simulink subsystem "VehicleEOMRef_Simp"  (R2022b)
settings: Solver=VariableStepAuto  StartTime=0.0  StopTime=10.0  RelTol=1e-3
undefined symbols (not defined in the file): Accel_bIi, Asensed_bIb, Newton, Omeg_BIb, OmegDtI_BIb, Pos_bii, Q_i2b, Raphson, SimIn, SimPar, Vel_bIi
libraries: libAxisTransformations x9, libMathOperations x9, libGeodesy x1, libKinematicalEquations x1
settings Model: Creator=drhill  LastModifiedBy=macheson
settings SolverCC: AlgebraicLoopSolver=TrustRegion
settings DebuggingCC: UnconnectedInputMsg=warning  UnconnectedOutputMsg=warning  UnconnectedLineMsg=warning  SFMachineParentedDataDiag=warning
settings ModelReferenceCC: EnableRefExpFcnMdlSchedulingChecks=on
settings RTWCC: DLArmComputeVersion=19.05

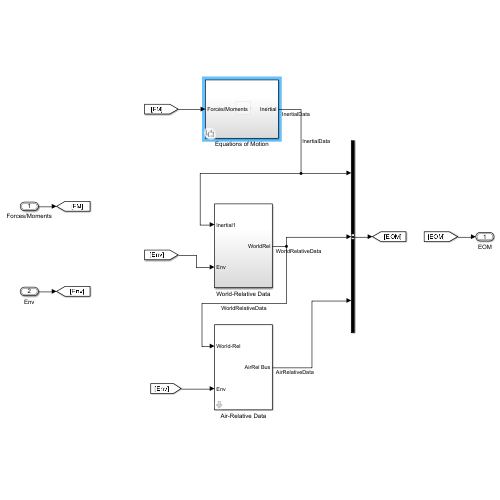
[thumbnail: Simulink's stored preview of the top-level diagram]
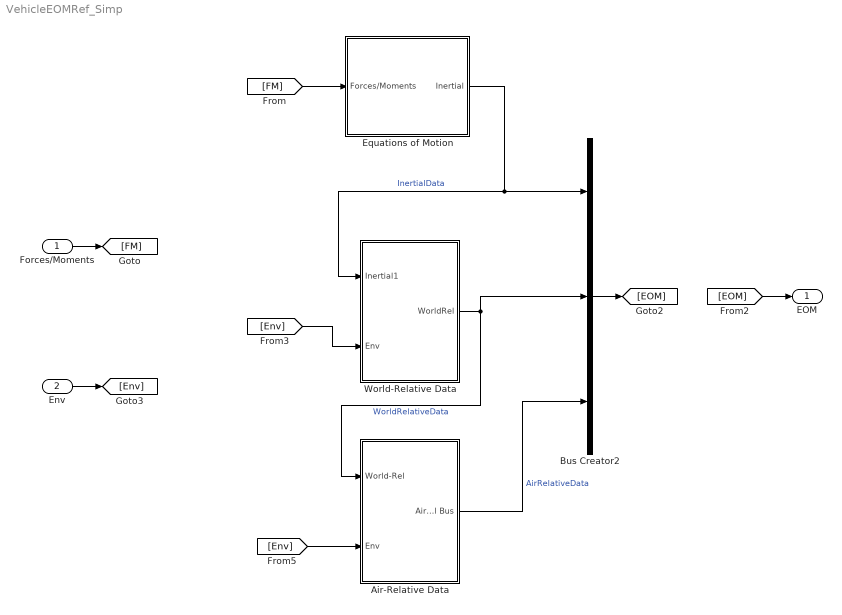
== system VehicleEOMRef_Simp ==
  Forces/Moments : Inport  OutDataTypeStr=Bus: ForceMomentBus
  Env : Inport  Port=2  OutDataTypeStr=Bus: EnvironmentBus
  Air-Relative Data : Subsystem  mask(Air-Relative Data (template)){}
      mask help: Template for common air-relative data.
  Bus Creator2 : BusCreator  Inputs=3  OutDataTypeStr=Bus: EomBus
  Equations of Motion : Subsystem  Variant=on  VariantControl=Variant1
  World-Relative Data : Subsystem
  EOM : Outport  OutDataTypeStr=Bus: EomBus
  wires:
  World-Relative Data/1(WorldRel) -> Air-Relative Data/1(World-Rel), Bus Creator2/2  "WorldRelativeData"
  Equations of Motion/1(Inertial) -> Bus Creator2/1, World-Relative Data/1(Inertial1)  "InertialData"
  Air-Relative Data/1(AirRel Bus) -> Bus Creator2/3  "AirRelativeData"
  [Env] -> Air-Relative Data/2(Env)
  [Env] -> World-Relative Data/2(Env)
  Env/1 -> [Env]
  [EOM] -> EOM/1
  Bus Creator2/1 -> [EOM]
  [FM] -> Equations of Motion/1(Forces/Moments)
  Forces/Moments/1 -> [FM]

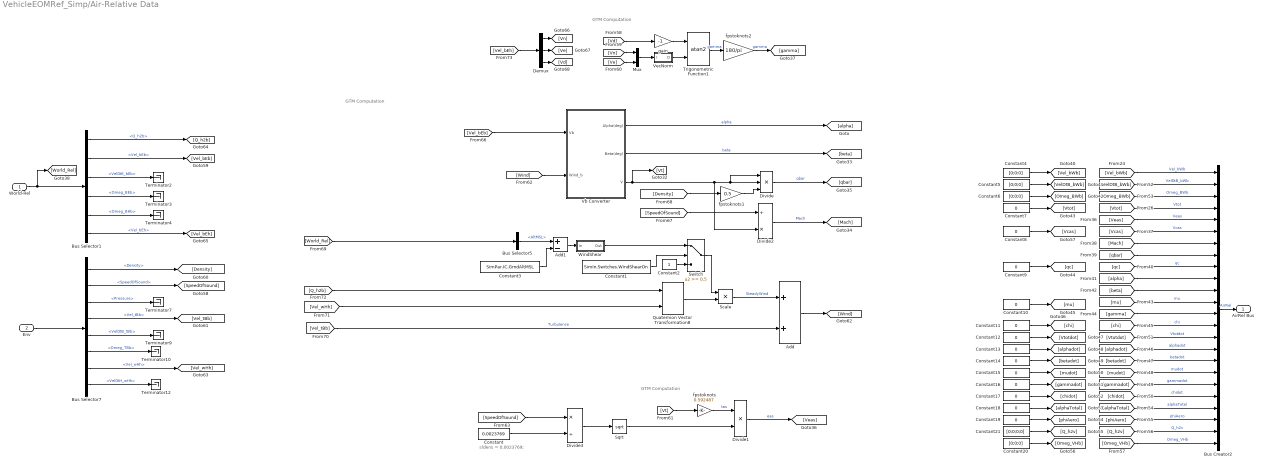
== system VehicleEOMRef_Simp/Air-Relative Data ==
  note: GTM Computation
  note: GTM Computation
  note: GTM Computation
  note: sldens = 0.0023769;
  World-Rel : Inport
  Env : Inport  Port=2
  Add : Sum
  Add1 : Sum  Inputs=+-
  Bus Creator2 : BusCreator  Inputs=24  OutDataTypeStr=Bus: AirRelBus
  Bus Selector1 : BusSelector  OutputSignals=Q_h2b,Vel_bEb,VelDtE_bEb,Omeg_BEb,Omeg_BHb,Vel_bEh
  Bus Selector5 : BusSelector  OutputSignals=AltMSL
  Bus Selector7 : BusSelector  OutputSignals=Atmosphere.Density,Atmosphere.SpeedOfSound,Atmosphere.Pressure,Turbulence.Vel_tBb,Turbulence.VelDtB_tBb,Turbulence.Omeg_TBb,Wind.Vel_wHh,Wind.VelDtH_wHh
  Constant : Constant  Value=0.0023769
  Constant1 : Constant  Value=SimIn.Switches.WindShearOn
  Constant{7..19} (13 alike) : Constant  Value=0
  Constant2 : Constant
  Constant{4..6,20} (4 alike) : Constant  Value=[0;0;0]
  Constant21 : Constant  Value=[0;0;0;0]
  Constant3 : Constant  Value=SimPar.IC.GrndAltMSL
  Demux : Demux  Outputs=3
  Divide : Product  Inputs=***
  Divide1 : Product
  Divide2 : Product  Inputs=/*
  Divide3 : Product  Inputs=*/
  Mux : Mux  Inputs=2
  Quaternion Vector Transformation8 : libAxisTransformations/Quaternion Vector Transformation  n=0
  Scale : Product  Inputs=**
  Sqrt : Sqrt
  Switch : Switch  Threshold=0.5  SaturateOnIntegerOverflow=off  InputSameDT=off
  Terminator{2..4,7,9..10,12} (7 alike) : Terminator
  Trigonometric Function1 : Trigonometry  Operator=atan2
  Vb Converter : Subsystem
  VecNorm : Subsystem
  WindShear : Subsystem
  fpstoknots : Gain  Gain=0.592487
  fpstoknots1 : Gain  Gain=0.5
  fpstoknots2 : Gain  Gain=180/pi
  gain : Gain  Gain=-1
  AirRel Bus : Outport
  wires:
  Demux/3 -> [Vd]
  Demux/2 -> [Ve]
  Demux/1 -> [Vn]
  [Vel_bEh] -> Demux/1
  Bus Selector1/6 -> [Vel_bEh]  "<Vel_bEh>"
  [Vel_bEb] -> Vb Converter/1(Vb)
  [Vel_wHh] -> Quaternion Vector Transformation8/2
  Bus Selector5/1 -> Add1/1  "<AltMSL>"
  [World_Rel] -> Bus Selector5/1
  Constant1/1 -> Switch/2
  Constant3/1 -> Add1/2
  Switch/1 -> Scale/1
  Scale/1 -> Add/1  "SteadyWind"
  Add/1 -> [Wind]
  Add1/1 -> WindShear/1(In)
  [Vel_tBb] -> Add/2  "Turbulence"
  Constant2/1 -> Switch/3
  WindShear/1(Out) -> Switch/1
  Quaternion Vector Transformation8/1 -> Scale/2
  [Q_h2b] -> Quaternion Vector Transformation8/1
  Sqrt/1 -> Divide1/2
  Divide3/1 -> Sqrt/1
  [SpeedOfSound] -> Divide3/1
  Constant/1 -> Divide3/2
  Constant8/1 -> [Vcas]
  Constant20/1 -> [Omeg_VHb]
  Constant21/1 -> [Q_h2v]
  Constant19/1 -> [phiAero]
  Constant18/1 -> [alphaTotal]
  Constant17/1 -> [chidot]
  Constant16/1 -> [gammadot]
  Constant15/1 -> [mudot]
  Constant14/1 -> [betadot]
  Constant13/1 -> [alphadot]
  Constant12/1 -> [Vtotdot]
  Constant11/1 -> [chi]
  Constant10/1 -> [mu]
  Constant9/1 -> [qc]
  Constant7/1 -> [Vtot]
  Constant6/1 -> [Omeg_BWb]
  Constant5/1 -> [VelDtB_bWb]
  Constant4/1 -> [Vel_bWb]
  [Vtot] -> Bus Creator2/4  "Vtot"
  Bus Creator2/1 -> AirRel Bus/1  "AirRel"
  [Vel_bWb] -> Bus Creator2/1  "Vel_bWb"
  [Veas] -> Bus Creator2/5  "Veas"
  [Vcas] -> Bus Creator2/6  "Vcas"
  [Mach] -> Bus Creator2/7
  [qbar] -> Bus Creator2/8
  [qc] -> Bus Creator2/9  "qc"
  [alpha] -> Bus Creator2/10
  [beta] -> Bus Creator2/11
  [mu] -> Bus Creator2/12  "mu"
  [gamma] -> Bus Creator2/13
  [chi] -> Bus Creator2/14  "chi"
  [alphadot] -> Bus Creator2/16  "alphadot"
  [betadot] -> Bus Creator2/17  "betadot"
  [mudot] -> Bus Creator2/18  "mudot"
  [gammadot] -> Bus Creator2/19  "gammadot"
  [chidot] -> Bus Creator2/20  "chidot"
  [Vtotdot] -> Bus Creator2/15  "Vtotdot"
  [VelDtB_bWb] -> Bus Creator2/2  "VelDtB_bWb"
  [Omeg_BWb] -> Bus Creator2/3  "Omeg_BWb"
  [alphaTotal] -> Bus Creator2/21  "alphaTotal"
  [phiAero] -> Bus Creator2/22  "phiAero"
  [Q_h2v] -> Bus Creator2/23  "Q_h2v"
  [Omeg_VHb] -> Bus Creator2/24  "Omeg_VHb"
  [Vd] -> gain/1
  gain/1 -> Trigonometric Function1/1
  Trigonometric Function1/1 -> fpstoknots2/1  "gamma"
  fpstoknots2/1 -> [gamma]  "gamma"
  [Vn] -> Mux/1
  Mux/1 -> VecNorm/1(I)
  [Ve] -> Mux/2
  VecNorm/1(O) -> Trigonometric Function1/2
  Vb Converter/3(V) -> Divide2/2, Divide/1, Divide/2, [Vt]
  [SpeedOfSound] -> Divide2/1
  [Density] -> fpstoknots1/1
  Vb Converter/1(Alpha(deg)) -> [alpha]  "alpha"
  Vb Converter/2(Beta(deg)) -> [beta]  "beta"
  Divide2/1 -> [Mach]  "Mach"
  [Wind] -> Vb Converter/2(Wind_b)
  Divide/1 -> [qbar]  "qbar"
  fpstoknots1/1 -> Divide/3
  fpstoknots/1 -> Divide1/1  "tas"
  [Vt] -> fpstoknots/1
  Divide1/1 -> [Veas]  "eas"
  World-Rel/1 -> [World_Rel], Bus Selector1/1
  Env/1 -> Bus Selector7/1
  Bus Selector1/1 -> [Q_h2b]  "<Q_h2b>"
  Bus Selector1/2 -> [Vel_bEb]  "<Vel_bEb>"
  Bus Selector1/3 -> Terminator2/1  "<VelDtE_bEb>"
  Bus Selector1/4 -> Terminator3/1  "<Omeg_BEb>"
  Bus Selector1/5 -> Terminator4/1  "<Omeg_BHb>"
  Bus Selector7/1 -> [Density]  "<Density>"
  Bus Selector7/2 -> [SpeedOfSound]  "<SpeedOfSound>"
  Bus Selector7/3 -> Terminator7/1  "<Pressure>"
  Bus Selector7/4 -> [Vel_tBb]  "<Vel_tBb>"
  Bus Selector7/5 -> Terminator9/1  "<VelDtB_tBb>"
  Bus Selector7/6 -> Terminator10/1  "<Omeg_TBb>"
  Bus Selector7/7 -> [Vel_wHh]  "<Vel_wHh>"
  Bus Selector7/8 -> Terminator12/1  "<VelDtH_wHh>"

== system VehicleEOMRef_Simp/Equations of Motion ==
  Forces/Moments : Inport
  SimpleEOM : Subsystem  VariantControl=GVS_EOM_TYPE_SIMPLE
  Inertial : Outport

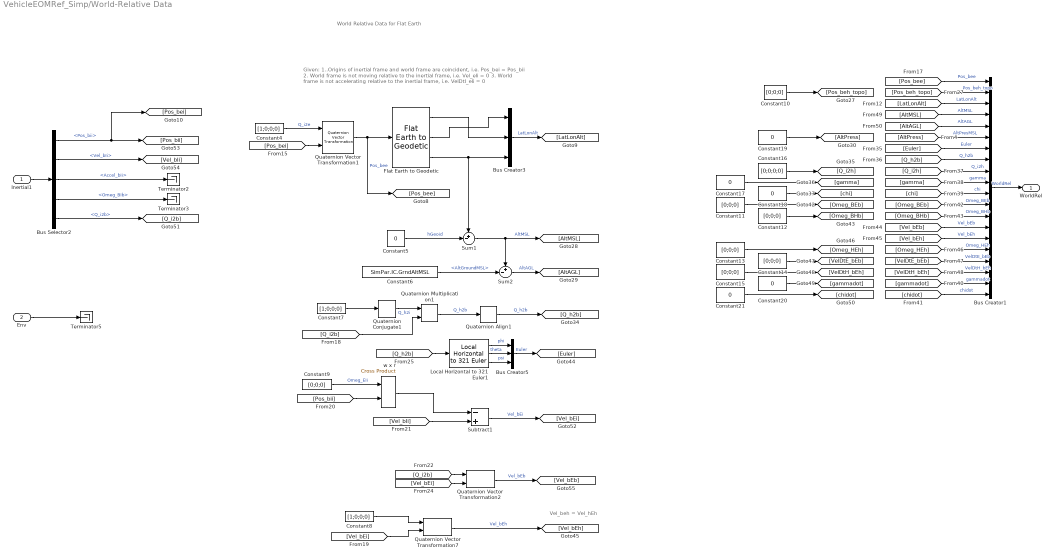
== system VehicleEOMRef_Simp/World-Relative Data ==
  note: Vel_beh = Vel_hEh
  note: World Relative Data for Flat Earth
  note: Given:
      | 1..Origins of inertial frame and world frame are coincident, i.e. Pos_bei = Pos_bii
      | 2. World frame is not moving relative to the inertial frame, i.e. Vel_eIi = 0
      | 3. World frame is not accelerating relative to the inertial frame, i.e. VelDtI_eIi = 0
  Inertial1 : Inport
  Env : Inport  Port=2
  Bus Creator1 : BusCreator  Inputs=20  OutDataTypeStr=Bus: WorldRelBus
  Bus Creator3 : BusCreator  Inputs=3  OutDataTypeStr=Bus: LatLonAltBus
  Bus Creator5 : BusCreator  Inputs=3  OutDataTypeStr=Bus: EulerBus
  Bus Selector2 : BusSelector  OutputSignals=Pos_bii,Vel_bIi,Accel_bIi,Omeg_BIb,Q_i2b
  Constant{10..15} (6 alike) : Constant  Value=[0;0;0]
  Constant16 : Constant  Value=[0;0;0;0]
  Constant{17..21} (5 alike) : Constant  Value=0
  Constant4 : Constant  Value=[1;0;0;0]  VectorParams1D=off
  Constant5 : Constant  Value=0  VectorParams1D=off
  Constant6 : Constant  Value=SimPar.IC.GrndAltMSL  VectorParams1D=off
  Constant7 : Constant  Value=[1;0;0;0]  VectorParams1D=off
  Constant8 : Constant  Value=[1;0;0;0]  VectorParams1D=off
  Constant9 : Constant  Value=[0;0;0]  VectorParams1D=off
  Flat Earth to Geodetic : libGeodesy/Flat Earth to Geodetic  lat=SimIn.IC.LatGeod  lon=SimIn.IC.Lon  a=SimIn.Environment.Earth.RadiusEquator  e=SimIn.Environment.Earth.Eccentricity
  Local Horizontal to 321 Euler1 : libKinematicalEquations/Local Horizontal to 321 Euler
  Quaternion Align1 : libMathOperations/Quaternion Align  n=0
  Quaternion Conjugate1 : libMathOperations/Quaternion Conjugate  n=0
  Quaternion Multiplication1 : libMathOperations/Quaternion Multiplication  n=0
  Quaternion Vector Transformation1 : libAxisTransformations/Quaternion Vector Transformation  n=0
  Quaternion Vector Transformation2 : libAxisTransformations/Quaternion Vector Transformation  n=0
  Quaternion Vector Transformation7 : libAxisTransformations/Quaternion Vector Transformation  n=0
  Subtract1 : Sum  Inputs=-+
  Sum1 : Sum  Inputs=+-|
  Sum2 : Sum  Inputs=+-|
  Terminator2 : Terminator
  Terminator3 : Terminator
  Terminator5 : Terminator
  w x r : libMathOperations/Cross Product
  WorldRel : Outport
  wires:
  [Q_h2b] -> Local Horizontal to 321 Euler1/1
  Local Horizontal to 321 Euler1/2 -> Bus Creator5/2  "theta"
  Bus Creator5/1 -> [Euler]  "Euler"
  Local Horizontal to 321 Euler1/1 -> Bus Creator5/1  "phi"
  Local Horizontal to 321 Euler1/3 -> Bus Creator5/3  "psi"
  [Vel_bEi] -> Quaternion Vector Transformation2/2
  [Q_i2b] -> Quaternion Vector Transformation2/1
  Quaternion Vector Transformation2/1 -> [Vel_bEb]  "Vel_bEb"
  Constant9/1 -> w x r/1  "Omeg_EIi"
  [Vel_bIi] -> Subtract1/2
  Subtract1/1 -> [Vel_bEi]  "Vel_bEi"
  [Pos_bii] -> w x r/2
  w x r/1 -> Subtract1/1
  Quaternion Vector Transformation7/1 -> [Vel_bEh]  "Vel_bEh"
  [Vel_bEi] -> Quaternion Vector Transformation7/2
  Constant8/1 -> Quaternion Vector Transformation7/1
  [Q_i2b] -> Quaternion Multiplication1/2
  Constant7/1 -> Quaternion Conjugate1/1
  Quaternion Multiplication1/1 -> Quaternion Align1/1  "Q_h2b"
  Quaternion Conjugate1/1 -> Quaternion Multiplication1/1  "Q_h2i"
  Quaternion Align1/1 -> [Q_h2b]  "Q_h2b"
  Constant21/1 -> [chidot]
  Constant20/1 -> [gammadot]
  Constant15/1 -> [VelDtH_bEh]
  Constant14/1 -> [VelDtE_bEb]
  Constant13/1 -> [Omeg_HEh]
  Constant12/1 -> [Omeg_BHb]
  Constant11/1 -> [Omeg_BEb]
  Constant18/1 -> [chi]
  Constant17/1 -> [gamma]
  Constant16/1 -> [Q_i2h]
  Constant19/1 -> [AltPress]
  Constant10/1 -> [Pos_beh_topo]
  Sum2/1 -> [AltAGL]  "AltAGL"
  Constant5/1 -> Sum1/2  "hGeoid"
  Flat Earth to Geodetic/3 -> Bus Creator3/3, Sum1/1
  Sum1/1 -> [AltMSL], Sum2/1  "AltMSL"
  Constant6/1 -> Sum2/2  "<AltGroundMSL>"
  Inertial1/1 -> Bus Selector2/1
  Bus Selector2/5 -> [Q_i2b]  "<Q_i2b>"
  Bus Selector2/2 -> [Vel_bIi]  "<Vel_bIi>"
  Bus Selector2/4 -> Terminator3/1  "<Omeg_BIb>"
  Bus Selector2/3 -> Terminator2/1  "<Accel_bIi>"
  Bus Selector2/1 -> [Pos_bei], [Pos_bii]  "<Pos_bii>"
  Bus Creator3/1 -> [LatLonAlt]  "LatLonAlt"
  Flat Earth to Geodetic/1 -> Bus Creator3/2
  Flat Earth to Geodetic/2 -> Bus Creator3/1
  [Pos_bei] -> Quaternion Vector Transformation1/2
  Quaternion Vector Transformation1/1 -> Flat Earth to Geodetic/1, [Pos_bee]  "Pos_bee"
  Constant4/1 -> Quaternion Vector Transformation1/1  "Q_i2e"
  Bus Creator1/1 -> WorldRel/1  "WorldRel"
  Env/1 -> Terminator5/1
  [AltMSL] -> Bus Creator1/4  "AltMSL"
  [AltAGL] -> Bus Creator1/5  "AltAGL"
  [AltPress] -> Bus Creator1/6  "AltPresMSL"
  [Pos_bee] -> Bus Creator1/1  "Pos_bee"
  [Pos_beh_topo] -> Bus Creator1/2  "Pos_beh_topo"
  [LatLonAlt] -> Bus Creator1/3  "LatLonAlt"
  [Euler] -> Bus Creator1/7  "Euler"
  [Q_h2b] -> Bus Creator1/8  "Q_h2b"
  [Q_i2h] -> Bus Creator1/9  "Q_i2h"
  [gamma] -> Bus Creator1/10  "gamma"
  [chi] -> Bus Creator1/11  "chi"
  [Omeg_BEb] -> Bus Creator1/12  "Omeg_BEb"
  [Omeg_BHb] -> Bus Creator1/13  "Omeg_BHb"
  [Vel_bEb] -> Bus Creator1/14  "Vel_bEb"
  [Vel_bEh] -> Bus Creator1/15  "Vel_bEh"
  [Omeg_HEh] -> Bus Creator1/16  "Omeg_HEh"
  [VelDtE_bEb] -> Bus Creator1/17  "VelDtE_bEb"
  [VelDtH_bEh] -> Bus Creator1/18  "VelDtH_bEh"
  [gammadot] -> Bus Creator1/19  "gammadot"
  [chidot] -> Bus Creator1/20  "chidot"

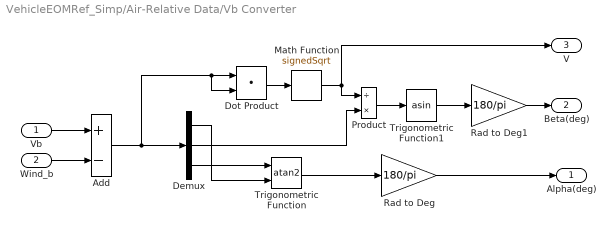
== system VehicleEOMRef_Simp/Air-Relative Data/Vb Converter ==
  Vb : Inport
  Wind_b : Inport  Port=2
  Add : Sum  Inputs=+-
  Demux : Demux  Outputs=3
      settings: DisplayOption=none
  Dot Product : DotProduct  OutDataTypeStr=Inherit: Inherit via internal rule
  Math Function : Sqrt  Operator=signedSqrt  AlgorithmType=Newton-Raphson
  Product : Product  Inputs=/*  SaturateOnIntegerOverflow=on  OutDataTypeStr=Inherit: Same as first input
  Rad to Deg : Gain  Gain=180/pi  SaturateOnIntegerOverflow=on  OutDataTypeStr=Inherit: Same as input  ParamDataTypeStr=Inherit: Same as input
  Rad to Deg1 : Gain  Gain=180/pi  SaturateOnIntegerOverflow=on  OutDataTypeStr=Inherit: Same as input  ParamDataTypeStr=Inherit: Same as input
  Trigonometric Function : Trigonometry  Operator=atan2
  Trigonometric Function1 : Trigonometry  Operator=asin
  Alpha(deg) : Outport  VectorParamsAs1DForOutWhenUnconnected=off
  Beta(deg) : Outport  Port=2  VectorParamsAs1DForOutWhenUnconnected=off
  V : Outport  Port=3  VectorParamsAs1DForOutWhenUnconnected=off
  wires:
  Add/1 -> Dot Product/2, Dot Product/1, Demux/1
  Vb/1 -> Add/1
  Wind_b/1 -> Add/2
  Demux/2 -> Product/2
  Math Function/1 -> V/1, Product/1
  Product/1 -> Trigonometric Function1/1
  Demux/3 -> Trigonometric Function/1
  Demux/1 -> Trigonometric Function/2
  Dot Product/1 -> Math Function/1
  Trigonometric Function/1 -> Rad to Deg/1
  Rad to Deg/1 -> Alpha(deg)/1
  Trigonometric Function1/1 -> Rad to Deg1/1
  Rad to Deg1/1 -> Beta(deg)/1

== system VehicleEOMRef_Simp/Air-Relative Data/VecNorm ==
  I : Inport
  Math Function2 : Sqrt  Operator=signedSqrt  AlgorithmType=Newton-Raphson
  Product : Product  RndMeth=Zero
  Sum of Elements : Sum  Inputs=+
  O : Outport  VectorParamsAs1DForOutWhenUnconnected=off
  wires:
  Math Function2/1 -> O/1
  I/1 -> Product/1, Product/2
  Product/1 -> Sum of Elements/1
  Sum of Elements/1 -> Math Function2/1

== system VehicleEOMRef_Simp/Air-Relative Data/WindShear ==
  note: ShearFactor = ln(h/.15) / ln(h/20), as per MIL-Spec: MIL-F-8785C
  In : Inport
  Constant2 : Constant  Value=log(20/.15);
  Divide : Product  Inputs=*/
  Gain : Gain  Gain=1/.15; %MILSpec constant
  Gain2 : Gain  Gain=1/1.8; % Scale to get unity gain@1000ft (instead of 20 ft)
  Math Function : Math  Operator=log  SignedPower=on
  Saturation : Saturate  UpperLimit=1000  LowerLimit=1
  Out : Outport  VectorParamsAs1DForOutWhenUnconnected=off
  wires:
  Gain2/1 -> Out/1
  Saturation/1 -> Gain/1
  Divide/1 -> Gain2/1
  Constant2/1 -> Divide/2
  Math Function/1 -> Divide/1
  In/1 -> Saturation/1
  Gain/1 -> Math Function/1

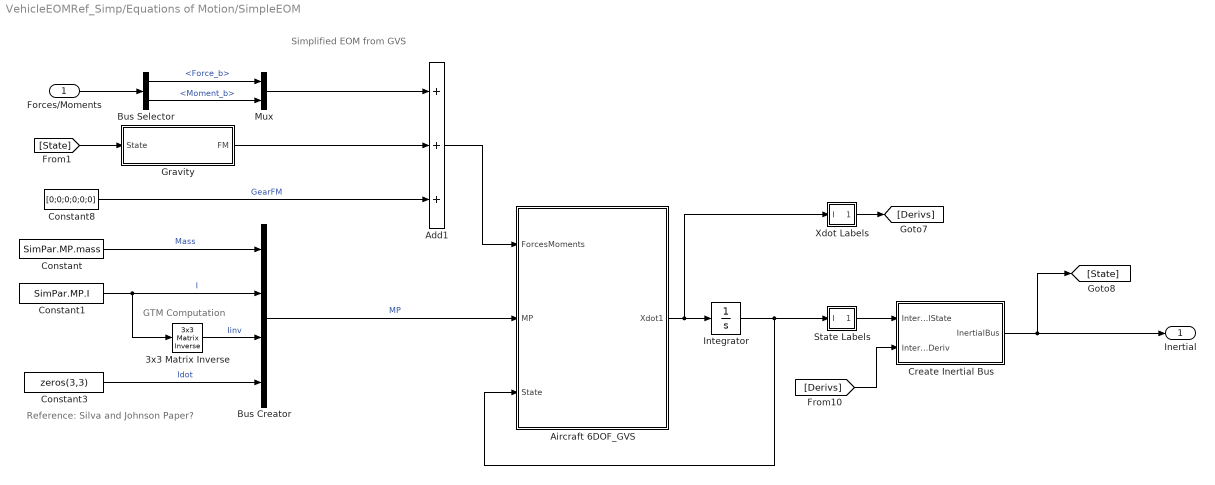
== system VehicleEOMRef_Simp/Equations of Motion/SimpleEOM ==
  note: GTM Computation
  note: Simplified EOM from GVS
  note: Reference: Silva and Johnson Paper?
  Forces/Moments : Inport
  3x3 Matrix Inverse : libMathOperations/3x3 Matrix Inverse
  Add1 : Sum  Inputs=+++
  Aircraft 6DOF_GVS : Subsystem
  Bus Creator : BusCreator  Inputs=4
  Bus Selector : BusSelector  OutputSignals=Total.Force_b,Total.Moment_b
  Constant : Constant  Value=SimPar.MP.mass
  Constant1 : Constant  Value=SimPar.MP.I
  Constant3 : Constant  Value=zeros(3,3)
  Constant8 : Constant  Value=[0;0;0;0;0;0]
  Create Inertial Bus : Subsystem
  Gravity : Subsystem
  Integrator : Integrator  InitialCondition=[SimPar.EOM.Vel_bEb; SimPar.EOM.Omeg_BIb; SimPar.EOM.Pos_bii; SimPar.EOM.Q_i2b]  LimitOutput=on  UpperSaturationLimit=[inf; inf; inf; 10; 10; 10; inf; inf; inf; 1; 1; 1; 1]  LowerSaturationLimit=-[inf; inf; inf; 10; 10; 10; inf; inf; inf; 1; 1; 1; 1]  ContinuousStateAttributes='EOMStates'
  Mux : Mux  Inputs=2
  State Labels : Subsystem
  Xdot Labels : Subsystem
  Inertial : Outport
  wires:
  3x3 Matrix Inverse/1 -> Bus Creator/3  "Iinv"
  Integrator/1 -> State Labels/1(I), Aircraft 6DOF_GVS/3(State)
  Mux/1 -> Add1/1
  Bus Selector/2 -> Mux/2  "<Moment_b>"
  Bus Selector/1 -> Mux/1  "<Force_b>"
  Constant3/1 -> Bus Creator/4  "Idot"
  Bus Creator/1 -> Aircraft 6DOF_GVS/2(MP)  "MP"
  Constant1/1 -> Bus Creator/2, 3x3 Matrix Inverse/1  "I"
  Constant/1 -> Bus Creator/1  "Mass"
  Xdot Labels/1(O) -> [Derivs]
  Aircraft 6DOF_GVS/1(Xdot1) -> Xdot Labels/1(I), Integrator/1
  Add1/1 -> Aircraft 6DOF_GVS/1(ForcesMoments)
  Gravity/1(FM) -> Add1/2
  Forces/Moments/1 -> Bus Selector/1
  State Labels/1(O) -> Create Inertial Bus/1(InternalState)
  Create Inertial Bus/1(InertialBus) -> Inertial/1, [State]
  [Derivs] -> Create Inertial Bus/2(InternalStateDeriv)
  [State] -> Gravity/1(State)
  Constant8/1 -> Add1/3  "GearFM"

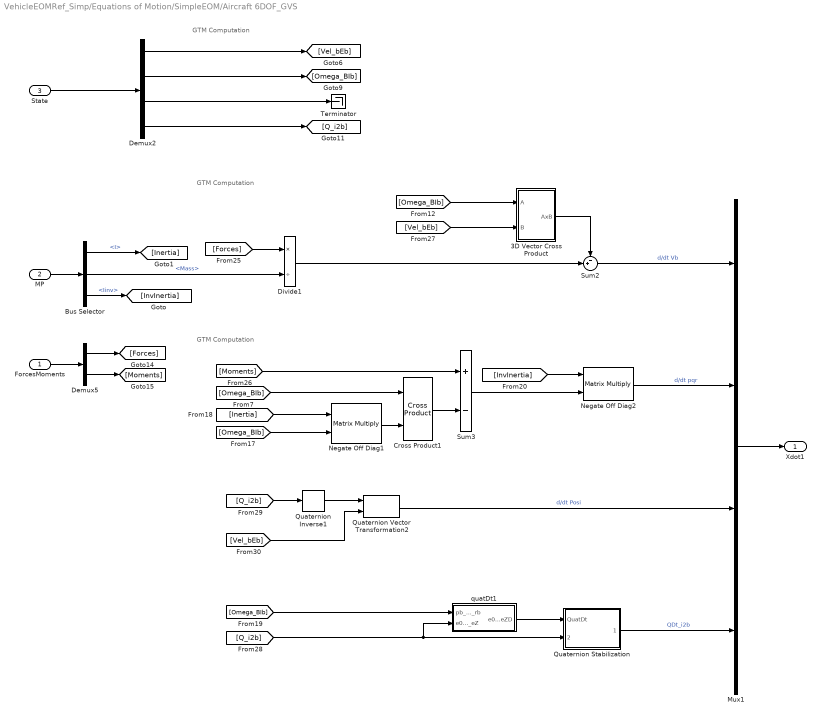
== system VehicleEOMRef_Simp/Equations of Motion/SimpleEOM/Aircraft 6DOF_GVS ==
  note: GTM Computation
  note: GTM Computation
  note: GTM Computation
  ForcesMoments : Inport
  MP : Inport  Port=2
  State : Inport  Port=3
  3D Vector Cross Product : Subsystem
  Bus Selector : BusSelector  OutputSignals=I,Mass,Iinv
  Cross Product1 : libMathOperations/Cross Product
  Demux2 : Demux  Outputs=[3 3 3 4]
  Demux5 : Demux  Outputs=[3 3]
  Divide1 : Product  Inputs=*/
  Mux1 : Mux
  Negate Off Diag1 : Product  Inputs=**  Multiplication=Matrix(*)
  Negate Off Diag2 : Product  Inputs=**  Multiplication=Matrix(*)
  Quaternion Stabilization : Subsystem
  Quaternion Inverse1 : libMathOperations/Quaternion Inverse  n=0
  Quaternion Vector Transformation2 : libAxisTransformations/Quaternion Vector Transformation  n=0
  Sum2 : Sum  Inputs=-+|  SaturateOnIntegerOverflow=on
  Sum3 : Sum  Inputs=+-  SaturateOnIntegerOverflow=on
  Terminator : Terminator
  quatDt1 : Subsystem  mask(QuatDt){}
      mask help:
      | Calculates rate of change of orientation
      | quaternion (i.e. d{e0,eX,eY,eZ}/dt) (1/sec)
      | based on body axis rotational rates {p,q,r}
      | (rad/sec), & current orientation quaternion
      | {e0,eX,eY,eZ} (non-dimensional).
      mask Help:
      | <h4>Block Description</h4><p>
      | 
      | Calculates rate of change of orientation quaternion (i.e. d{e<sub>0</sub>,e<sub>X</sub>,e<sub>Y</sub>,e<sub>Z</sub>}/dt) (1/sec)
      | <br />based on body axis rotational rates {p,q,r} (rad/sec),
      | <br />&amp; current orientation quaternion {e<sub>0</sub>,e<sub>X</sub>,e<sub>Y</sub>,e<sub>Z</sub>} (non-dimensional).
      | 
      | </p><p>The block input and output contain more than one signal as described below.</p>
      | 
      | <table><thead><strong>Reference Documents</strong></thead>
      | <tr>
      | <td align="center" width="45">
      | <cite><strong>Review of Attitude Representations
      | <br />Used for Aircraft Kinematics</strong>
      | <br />Journal of Aircraft
      | <br />Vol. 38, No. 4, July-August 2001
      | 
      | <!---
      | <br />W.F. Phillips and C.E. Hailey
      | <br />Utah State University, Logan, UT  84322
      | <br />and
      | <br />G.A. Gebert
      | <br />Sverdrup Technology, Inc.
      | <br />Eglin AFB, FL 32542
      | --->
      | 
      | </cite></td>
      | <td width="5%"></td>
      | <td align="center" width="50%"><cite><strong>Recommended Practice for Atmospheric and
      | <br />Space Flight Vehicle Coordinate Systems</strong>
      | <br />ANSI&#47;AIAA   R-004-1992
      | <br />American National Standard Institute
      | <br />sponsored by
      | <br />American Institute of
      | <br />Aeronautics &amp; Astronautics</cite></td>
      | </tr>
      | <tr><td align="center" width="45%"><strong>Equation:
      | </strong> (31)</td>
      | <td width="5%"></td>
      | <td align="center" width="50%"><strong>
      | Sign convention from:</strong> (1.4.6)</td></tr>
      | </table>
      | 
      | <!---Implemented by David Christhilf
      |         Lockheed - Martin Engr. &amp; Sc. Co.
      |         Langley Program Office
      |         supporting NASA-Langley Research Center
      |         2002-08-21
      |         d.m.christhilf@larc.nasa.gov--->
      | 
      | <h4>Block Vector Input Port #1 - Body Axis Rotational Rates (rad/sec)</h4>
      | <table><tr>
      | <td><ul>
      |    <li>pb_rps</li>
      |    <li>qb_rps</li>
      |    <li>rb_rps</li>
      | </ul></td>
      | <td><dl><br />
      |    <dd>roll rate</dd>
      |    <dd>pitch rate</dd>
      |    <dd>yaw rate</dd>
      | </dl></td>
      | <td align="center"><dl><br />
      |    <dd>(+rt_wing_dn)</dd>
      |    <dd>(+nose_up)</dd>
      |    <dd>(+nose_rt)</dd>
      | </dl></td>
      | </tr></table>
      | 
      | <h4>Block Vector Input Port #2 - Orientation Quaternion (non-dimensional)</h4>
      | <ul>
      |    <li>e<sub>0</sub></li>
      |    <li>e<sub>X</sub></li>
      |    <li>e<sub>Y</sub></li>
      |    <li>e<sub>Z</sub></li>
      | </ul>
      | 
      | <h4>Block Vector Output - Time Derivative of Orientation Quaternion (1/sec)</h4>
      | <ul>
      |    <li>e0dt</li>
      |    <li>eXdt</li>
      |    <li>eYdt</li>
      |    <li>eZdt</li>
      | </ul>
      mask Display: disp('QuatDt')
  Xdot1 : Outport  VectorParamsAs1DForOutWhenUnconnected=off
  wires:
  [Forces] -> Divide1/1
  Bus Selector/3 -> [InvInertia]  "<Iinv>"
  Bus Selector/1 -> [Inertia]  "<I>"
  MP/1 -> Bus Selector/1
  [Omega_BIb] -> 3D Vector Cross Product/1(A)
  Mux1/1 -> Xdot1/1
  Demux2/2 -> [Omega_BIb]
  Demux2/4 -> [Q_i2b]
  Demux2/3 -> Terminator/1
  Cross Product1/1 -> Sum3/2
  Sum3/1 -> Negate Off Diag2/2
  [Omega_BIb] -> Negate Off Diag1/2
  [Vel_bEb] -> 3D Vector Cross Product/2(B)
  Negate Off Diag1/1 -> Cross Product1/2
  Demux2/1 -> [Vel_bEb]
  3D Vector Cross Product/1(AxB) -> Sum2/1
  [InvInertia] -> Negate Off Diag2/1
  Negate Off Diag2/1 -> Mux1/2  "d/dt pqr"
  State/1 -> Demux2/1
  Bus Selector/2 -> Divide1/2  "<Mass>"
  [Omega_BIb] -> Cross Product1/1
  Divide1/1 -> Sum2/2
  [Inertia] -> Negate Off Diag1/1
  Sum2/1 -> Mux1/1  "d/dt Vb"
  [Moments] -> Sum3/1
  ForcesMoments/1 -> Demux5/1
  Demux5/2 -> [Moments]
  Demux5/1 -> [Forces]
  quatDt1/1(e0D_eXD_eYD_eZD) -> Quaternion Stabilization/1(QuatDt)
  [Q_i2b] -> quatDt1/2(e0_eX_eY_eZ), Quaternion Stabilization/2(Quat_i2b)
  Quaternion Stabilization/1(qdot out) -> Mux1/4  "QDt_i2b"
  [Omega_BIb] -> quatDt1/1(pb_qb_rb)
  Quaternion Inverse1/1 -> Quaternion Vector Transformation2/1
  [Q_i2b] -> Quaternion Inverse1/1
  [Vel_bEb] -> Quaternion Vector Transformation2/2
  Quaternion Vector Transformation2/1 -> Mux1/3  "d/dt Posi"

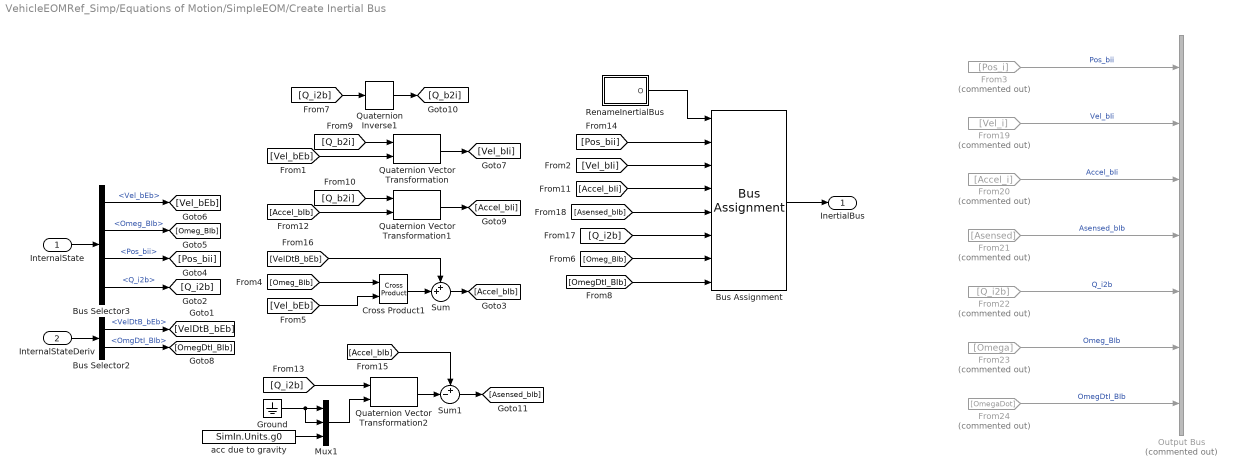
== system VehicleEOMRef_Simp/Equations of Motion/SimpleEOM/Create Inertial Bus ==
  InternalState : Inport
  InternalStateDeriv : Inport  Port=2
  Bus Assignment : BusAssignment  AssignedSignals=Pos_bii,Vel_bIi,Accel_bIi,Asensed_bIb,Q_i2b,Omeg_BIb,OmegDtI_BIb
  Bus Selector2 : BusSelector  OutputSignals=VelDtB_bEb,OmgDtI_BIb
  Bus Selector3 : BusSelector  OutputSignals=Vel_bEb,Omeg_BIb,Pos_bii,Q_i2b
  Cross Product1 : libMathOperations/Cross Product
  From19 : From  Commented=on  GotoTag=Vel_i
  From20 : From  Commented=on  GotoTag=Accel_i
  From21 : From  Commented=on  GotoTag=Asensed
  From22 : From  Commented=on  GotoTag=Q_i2b
  From23 : From  Commented=on  GotoTag=Omega
  From24 : From  Commented=on  GotoTag=OmegaDot
  From3 : From  Commented=on  GotoTag=Pos_i
  Ground : Ground
  Mux1 : Mux  Inputs=3
  Output Bus : BusCreator  Commented=on  Inputs=7
  Quaternion Inverse1 : libMathOperations/Quaternion Inverse  n=0
  Quaternion Vector Transformation : libAxisTransformations/Quaternion Vector Transformation  n=0
  Quaternion Vector Transformation1 : libAxisTransformations/Quaternion Vector Transformation  n=0
  Quaternion Vector Transformation2 : libAxisTransformations/Quaternion Vector Transformation  n=0
  RenameInertialBus : Subsystem
  Sum : Sum  Inputs=++|  SaturateOnIntegerOverflow=on
  Sum1 : Sum  Inputs=+-|  SaturateOnIntegerOverflow=on
  acc due to gravity : Constant  Value=SimIn.Units.g0
  InertialBus : Outport  VectorParamsAs1DForOutWhenUnconnected=off
  wires:
  From20/1 -> Output Bus/3  "Accel_bIi"
  From23/1 -> Output Bus/6  "Omeg_BIb"
  From21/1 -> Output Bus/4  "Asensed_bIb"
  From24/1 -> Output Bus/7  "OmegDtI_BIb"
  From3/1 -> Output Bus/1  "Pos_bii"
  From19/1 -> Output Bus/2  "Vel_bIi"
  From22/1 -> Output Bus/5  "Q_i2b"
  RenameInertialBus/1(O) -> Bus Assignment/1
  [Vel_bIi] -> Bus Assignment/3
  [Asensed_bIb] -> Bus Assignment/5
  [Accel_bIi] -> Bus Assignment/4
  [Pos_bii] -> Bus Assignment/2
  Bus Assignment/1 -> InertialBus/1
  InternalStateDeriv/1 -> Bus Selector2/1
  [Q_b2i] -> Quaternion Vector Transformation/1
  InternalState/1 -> Bus Selector3/1
  Bus Selector3/4 -> [Q_i2b]  "<Q_i2b>"
  Bus Selector3/3 -> [Pos_bii]  "<Pos_bii>"
  Bus Selector3/2 -> [Omeg_BIb]  "<Omeg_BIb>"
  Bus Selector3/1 -> [Vel_bEb]  "<Vel_bEb>"
  [Vel_bEb] -> Quaternion Vector Transformation/2
  Quaternion Vector Transformation/1 -> [Vel_bIi]
  Bus Selector2/1 -> [VelDtB_bEb]  "<VelDtB_bEb>"
  Bus Selector2/2 -> [OmegDtI_BIb]  "<OmgDtI_BIb>"
  [Q_i2b] -> Quaternion Inverse1/1
  Quaternion Inverse1/1 -> [Q_b2i]
  Quaternion Vector Transformation1/1 -> [Accel_bIi]
  [Q_b2i] -> Quaternion Vector Transformation1/1
  [Q_i2b] -> Bus Assignment/6
  [Omeg_BIb] -> Bus Assignment/7
  [OmegDtI_BIb] -> Bus Assignment/8
  [Vel_bEb] -> Cross Product1/2
  [Omeg_BIb] -> Cross Product1/1
  [VelDtB_bEb] -> Sum/1
  Cross Product1/1 -> Sum/2
  Sum/1 -> [Accel_bIb]
  [Accel_bIb] -> Quaternion Vector Transformation1/2
  acc due to gravity/1 -> Mux1/3
  Ground/1 -> Mux1/2, Mux1/1
  Mux1/1 -> Quaternion Vector Transformation2/2
  [Q_i2b] -> Quaternion Vector Transformation2/1
  Quaternion Vector Transformation2/1 -> Sum1/2
  [Accel_bIb] -> Sum1/1
  Sum1/1 -> [Asensed_bIb]

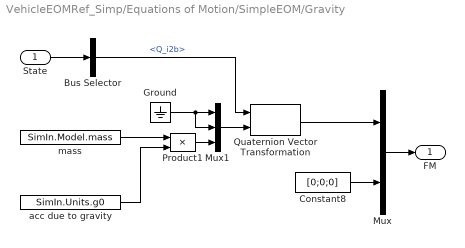
== system VehicleEOMRef_Simp/Equations of Motion/SimpleEOM/Gravity ==
  State : Inport
  Bus Selector : BusSelector  OutputSignals=Q_i2b
  Constant8 : Constant  Value=[0;0;0]
  Ground : Ground
  Mux : Mux  Inputs=[3 3]
  Mux1 : Mux  Inputs=3
  Product1 : Product  RndMeth=Zero
  Quaternion Vector Transformation : libAxisTransformations/Quaternion Vector Transformation  n=0
  acc due to gravity : Constant  Value=SimIn.Units.g0
  mass : Constant  Value=SimIn.Model.mass
  FM : Outport  VectorParamsAs1DForOutWhenUnconnected=off
  wires:
  acc due to gravity/1 -> Product1/2
  Constant8/1 -> Mux/2
  Product1/1 -> Mux1/3
  Ground/1 -> Mux1/2, Mux1/1
  Mux1/1 -> Quaternion Vector Transformation/2
  Mux/1 -> FM/1
  Quaternion Vector Transformation/1 -> Mux/1
  mass/1 -> Product1/1
  State/1 -> Bus Selector/1
  Bus Selector/1 -> Quaternion Vector Transformation/1  "<Q_i2b>"

== system VehicleEOMRef_Simp/Equations of Motion/SimpleEOM/State Labels ==
  I : Inport
  Bus Creator : BusCreator  Inputs=4
  Demux : Demux  Outputs=[3 3 3 4]
      settings: DisplayOption=none
  Reshape{1..3,5} (4 alike) : Reshape  OutputDimensionality=Column vector (2-D)
  O : Outport  VectorParamsAs1DForOutWhenUnconnected=off
  wires:
  Demux/3 -> Reshape3/1  "Pos_bii"
  Reshape3/1 -> Bus Creator/3  "Pos_bii"
  Demux/2 -> Reshape2/1  "Omeg_BIb"
  Reshape2/1 -> Bus Creator/2  "Omeg_BIb"
  Demux/1 -> Reshape1/1  "Vel_bEb"
  Reshape1/1 -> Bus Creator/1  "Vel_bEb"
  I/1 -> Demux/1
  Bus Creator/1 -> O/1
  Demux/4 -> Reshape5/1  "Q_i2b"
  Reshape5/1 -> Bus Creator/4  "Q_i2b"

== system VehicleEOMRef_Simp/Equations of Motion/SimpleEOM/Xdot Labels ==
  I : Inport
  Bus Creator : BusCreator  Inputs=4
  Demux : Demux  Outputs=[3 3 3 4]
      settings: DisplayOption=none
  O : Outport  VectorParamsAs1DForOutWhenUnconnected=off
  wires:
  Bus Creator/1 -> O/1
  I/1 -> Demux/1
  Demux/1 -> Bus Creator/1  "VelDtB_bEb"
  Demux/2 -> Bus Creator/2  "OmgDtI_BIb"
  Demux/3 -> Bus Creator/3  "PosDtI_bii"
  Demux/4 -> Bus Creator/4  "QDt_i2b"

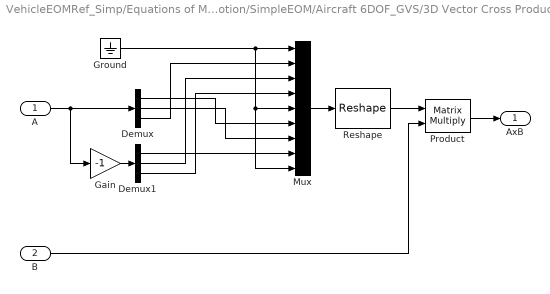
== system VehicleEOMRef_Simp/Equations of Motion/SimpleEOM/Aircraft 6DOF_GVS/3D Vector Cross Product ==
  A : Inport
  B : Inport  Port=2
  Demux : Demux  Outputs=3
      settings: DisplayOption=none
  Demux1 : Demux  Outputs=3
      settings: DisplayOption=none
  Gain : Gain  Gain=-1  SaturateOnIntegerOverflow=on  OutDataTypeStr=Inherit: Same as input  ParamDataTypeStr=Inherit: Same as input
  Ground : Ground
  Mux : Mux  Inputs=9
  Product : Product  Multiplication=Matrix(*)  SaturateOnIntegerOverflow=on  OutDataTypeStr=Inherit: Same as first input
  Reshape : Reshape  OutputDimensionality=Customize  OutputDimensions=[3,3]
  AxB : Outport  VectorParamsAs1DForOutWhenUnconnected=off
  wires:
  A/1 -> Demux/1, Gain/1
  Product/1 -> AxB/1
  Ground/1 -> Mux/1, Mux/5, Mux/9
  Gain/1 -> Demux1/1
  Demux/3 -> Mux/2
  Demux1/2 -> Mux/3
  Demux1/3 -> Mux/4
  Demux/1 -> Mux/6
  Demux/2 -> Mux/7
  Demux1/1 -> Mux/8
  Mux/1 -> Reshape/1
  Reshape/1 -> Product/1
  B/1 -> Product/2

== system VehicleEOMRef_Simp/Equations of Motion/SimpleEOM/Aircraft 6DOF_GVS/Quaternion Stabilization ==
  QuatDt : Inport  PortDimensions=[4,1]
  Quat_i2b : Inport  Port=2  PortDimensions=[4,1]
  Product : Product  InputSameDT=on  SaturateOnIntegerOverflow=on  OutDataTypeStr=Inherit: Same as first input
  Stab_gain : Subsystem
  Sum1 : Sum  Inputs=-+  InputSameDT=on  SaturateOnIntegerOverflow=on  OutDataTypeStr=Inherit: Same as first input
  qdot out : Outport  PortDimensions=[4,1]  VectorParamsAs1DForOutWhenUnconnected=off
  wires:
  QuatDt/1 -> Sum1/2
  Sum1/1 -> qdot out/1
  Quat_i2b/1 -> Product/2, Stab_gain/1(Quat_i2b)
  Stab_gain/1(stabilization_gain) -> Product/1
  Product/1 -> Sum1/1

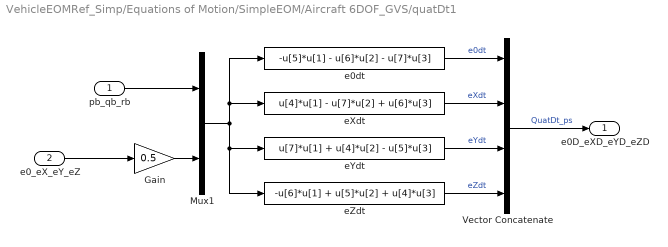
== system VehicleEOMRef_Simp/Equations of Motion/SimpleEOM/Aircraft 6DOF_GVS/quatDt1 ==
  pb_qb_rb : Inport  PortDimensions=[3,1]
  e0_eX_eY_eZ : Inport  Port=2  PortDimensions=[4,1]
  Gain : Gain  Gain=0.5  SaturateOnIntegerOverflow=on  OutDataTypeStr=Inherit: Same as input  ParamDataTypeStr=Inherit: Same as input
  Mux1 : Mux  Inputs=[3 4]
  Vector Concatenate : Concatenate  NumInputs=4  Mode=Multidimensional array
  e0dt : Fcn  Expr=-u[5]*u[1] - u[6]*u[2] - u[7]*u[3]
  eXdt : Fcn  Expr=u[4]*u[1] - u[7]*u[2] + u[6]*u[3]
  eYdt : Fcn  Expr=u[7]*u[1] + u[4]*u[2] - u[5]*u[3]
  eZdt : Fcn  Expr=-u[6]*u[1] + u[5]*u[2] + u[4]*u[3]
  e0D_eXD_eYD_eZD : Outport  PortDimensions=[4,1]  VectorParamsAs1DForOutWhenUnconnected=off
  wires:
  Mux1/1 -> eZdt/1, eYdt/1, e0dt/1, eXdt/1
  eZdt/1 -> Vector Concatenate/4  "eZdt"
  pb_qb_rb/1 -> Mux1/1
  Gain/1 -> Mux1/2
  eYdt/1 -> Vector Concatenate/3  "eYdt"
  eXdt/1 -> Vector Concatenate/2  "eXdt"
  e0dt/1 -> Vector Concatenate/1  "e0dt"
  Vector Concatenate/1 -> e0D_eXD_eYD_eZD/1  "QuatDt_ps"
  e0_eX_eY_eZ/1 -> Gain/1

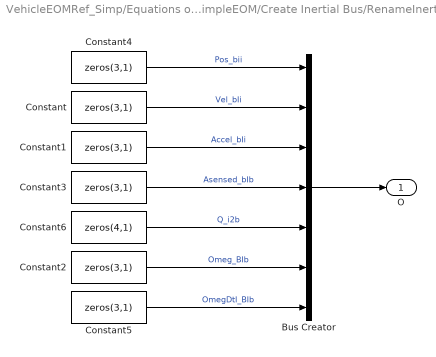
== system VehicleEOMRef_Simp/Equations of Motion/SimpleEOM/Create Inertial Bus/RenameInertialBus ==
  Bus Creator : BusCreator  Inputs=7  OutDataTypeStr=Bus: InertialBus
  Constant{,1..5} (6 alike) : Constant  Value=zeros(3,1)  VectorParams1D=off
  Constant6 : Constant  Value=zeros(4,1)  VectorParams1D=off
  O : Outport  VectorParamsAs1DForOutWhenUnconnected=off
  wires:
  Constant3/1 -> Bus Creator/4  "Asensed_bIb"
  Constant1/1 -> Bus Creator/3  "Accel_bIi"
  Constant/1 -> Bus Creator/2  "Vel_bIi"
  Constant4/1 -> Bus Creator/1  "Pos_bii"
  Bus Creator/1 -> O/1
  Constant5/1 -> Bus Creator/7  "OmegDtI_BIb"
  Constant2/1 -> Bus Creator/6  "Omeg_BIb"
  Constant6/1 -> Bus Creator/5  "Q_i2b"

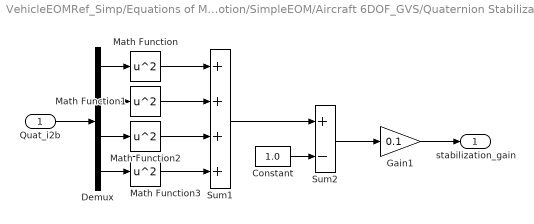
== system VehicleEOMRef_Simp/Equations of Motion/SimpleEOM/Aircraft 6DOF_GVS/Quaternion Stabilization/Stab_gain ==
  Quat_i2b : Inport  PortDimensions=[4,1]
  Constant : Constant  Value=1.0
  Demux : Demux
      settings: DisplayOption=none
  Gain1 : Gain  Gain=0.1  SaturateOnIntegerOverflow=on  OutDataTypeStr=Inherit: Same as input  ParamDataTypeStr=Inherit: Same as input
  Math Function{,1..3} (4 alike) : Math  Operator=square  SignedPower=on
  Sum1 : Sum  Inputs=4  SaturateOnIntegerOverflow=on
  Sum2 : Sum  Inputs=+-  SaturateOnIntegerOverflow=on
  stabilization_gain : Outport  PortDimensions=1  VectorParamsAs1DForOutWhenUnconnected=off
  wires:
  Sum1/1 -> Sum2/1
  Math Function/1 -> Sum1/1
  Math Function1/1 -> Sum1/2
  Math Function2/1 -> Sum1/3
  Math Function3/1 -> Sum1/4
  Constant/1 -> Sum2/2
  Sum2/1 -> Gain1/1
  Gain1/1 -> stabilization_gain/1
  Demux/1 -> Math Function/1
  Demux/2 -> Math Function1/1
  Demux/3 -> Math Function2/1
  Demux/4 -> Math Function3/1
  Quat_i2b/1 -> Demux/1
